simulink model "FM_Broadcast_Transmitter"  (R2022a)
settings: Solver=FixedStepDiscrete  StartTime=0.0  StopTime=inf  RelTol=1e-3
libraries: dspsrcs4 x2, dspsigops x2, matrix_library x2, commsynccomp2 x1, dspvision x1
settings Model: Creator=vovan  LastModifiedBy=vovan

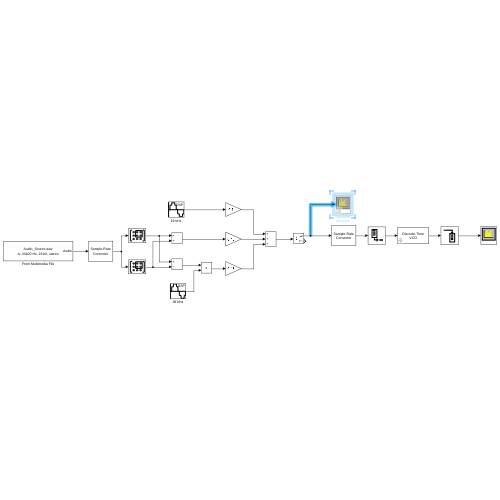
[thumbnail: Simulink's stored preview of the top-level diagram]
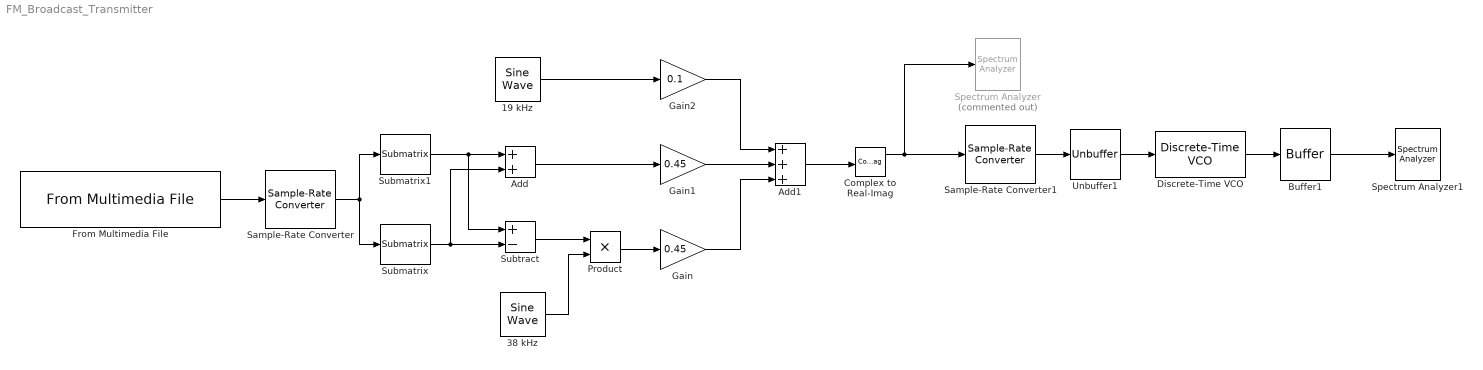
== system FM_Broadcast_Transmitter ==
  19 kHz : dspsrcs4/Sine Wave  Amplitude=1  Frequency=19e3  Phase=0  SampleMode=Discrete  OutComplex=Complex  CompMethod=Trigonometric fcn  TableSize=Speed  SampleTime=1/(44100*5)  SamplesPerFrame=512*5  ResetState=Restart at time zero  OutputFrames=off  dataType=double  wordLen=16  udDataType=sfix(16)  fracBitsMode=Best precision  numFracBits=15  OutDataTypeStr=double  LastOutDataTypeStr=double
  38 kHz : dspsrcs4/Sine Wave  Amplitude=1  Frequency=38e3  Phase=0  SampleMode=Discrete  OutComplex=Complex  CompMethod=Trigonometric fcn  TableSize=Speed  SampleTime=1/(44100*5)  SamplesPerFrame=512*5  ResetState=Restart at time zero  OutputFrames=off  dataType=double  wordLen=16  udDataType=sfix(16)  fracBitsMode=Best precision  numFracBits=15  OutDataTypeStr=double  LastOutDataTypeStr=double
  Add : Sum
  Add1 : Sum  Inputs=+++
  Buffer1 : Buffer  N=512*5  OutputFrames=off
  Complex to Real-Imag : ComplexToRealImag
  Discrete-Time VCO : commsynccomp2/Discrete-Time VCO  Ac=1  Fc=0  Kc=75e3  Ph=0  ts=-1
      settings: SourceProductBaseCode=CM
  From Multimedia File : dspvision/From Multimedia File  inputFilename=wav/Audio_Source.wav  readRange=[1 Inf]  loop=on  numPlays=inf  outputStreams=Audio only  videoDataType=single  audioDataType=double  inheritSampleTime=on  userDefinedSampleTime=1/30  noAudioOutput=off  isIntensityVideo=off  fourcc=RGB  colorVideoFormat=Separate color signals  outputEOF=off  dataOrg=Column-major  audioFrameSize=512  computeAudioFrameSize=off  outSamplingMode=Sample based
  Gain : Gain  Gain=0.45
  Gain1 : Gain  Gain=0.45
  Gain2 : Gain  Gain=0.1
  Product : Product
  Sample-Rate Converter : dspsigops/Sample-Rate Converter  InputSampleRate=44100  OutputSampleRate=5*44100  OutputRateTolerance=0  Bandwidth=40e3  StopbandAttenuation=80  SimulateUsing=Code generation
      settings: SourceProductBaseCode=DS
  Sample-Rate Converter1 : dspsigops/Sample-Rate Converter  InputSampleRate=5*44100  OutputSampleRate=25*44100  OutputRateTolerance=0  Bandwidth=110e3  StopbandAttenuation=80  SimulateUsing=Code generation
      settings: SourceProductBaseCode=DS
  Spectrum Analyzer : SpectrumAnalyzer  Commented=on
  Spectrum Analyzer1 : SpectrumAnalyzer
  Submatrix : matrix_library/Submatrix  RowSpan=All rows  RowStartMode=First  RowStartIndex=1  RowEndMode=Last  RowEndIndex=1  ColSpan=Range of columns  ColStartMode=Last  ColStartIndex=1  ColEndMode=Index  ColEndIndex=1
      settings: SourceProductBaseCode=SL
  Submatrix1 : matrix_library/Submatrix  RowSpan=All rows  RowStartMode=First  RowStartIndex=1  RowEndMode=Last  RowEndIndex=1  ColSpan=Range of columns  ColStartMode=First  ColStartIndex=1  ColEndMode=Index  ColEndIndex=1
      settings: SourceProductBaseCode=SL
  Subtract : Sum  Inputs=+-
  Unbuffer1 : Unbuffer
  wires:
  From Multimedia File/1 -> Sample-Rate Converter/1
  Unbuffer1/1 -> Discrete-Time VCO/1
  Buffer1/1 -> Spectrum Analyzer1/1
  Discrete-Time VCO/1 -> Buffer1/1
  Sample-Rate Converter/1 -> Submatrix/1, Submatrix1/1
  Submatrix/1 -> Add/2, Subtract/2
  Submatrix1/1 -> Subtract/1, Add/1
  19 kHz/1 -> Gain2/1
  38 kHz/1 -> Product/2
  Subtract/1 -> Product/1
  Product/1 -> Gain/1
  Add/1 -> Gain1/1
  Gain1/1 -> Add1/2
  Gain2/1 -> Add1/1
  Gain/1 -> Add1/3
  Add1/1 -> Complex to Real-Imag/1
  Complex to Real-Imag/1 -> Sample-Rate Converter1/1, Spectrum Analyzer/1
  Sample-Rate Converter1/1 -> Unbuffer1/1
